simulink model "DYN_04"  (R2018b)
settings: Solver=FixedStepAuto  StartTime=0.0  StopTime=30  FixedStep=0.01  RelTol=1e-3
(part 1 of 14)
settings Model: Creator=TMP  LastModifiedBy=TMP
settings DataIOCC: ReturnWorkspaceOutputs=on

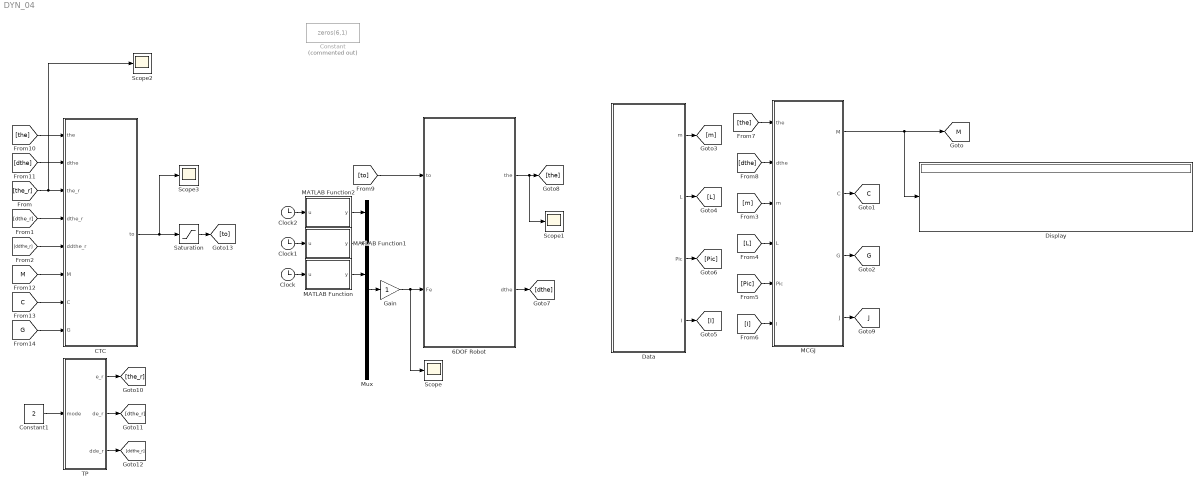
== system DYN_04 ==
  6DOF Robot : Subsystem
  CTC : MATLAB Function  TreatAsAtomicUnit=on
  Clock : Clock
  Clock1 : Clock
  Clock2 : Clock
  Constant : Constant  Commented=on  Value=zeros(6,1)
  Constant1 : Constant  Value=2
  Data : MATLAB Function  TreatAsAtomicUnit=on
  Display : Display
  Gain : Gain
  MATLAB Function : MATLAB Function  TreatAsAtomicUnit=on
  MATLAB Function1 : MATLAB Function  TreatAsAtomicUnit=on
  MATLAB Function2 : MATLAB Function  TreatAsAtomicUnit=on
  MCGJ : MATLAB Function  TreatAsAtomicUnit=on
  Mux : Mux  Inputs=6
  Saturation : Saturate  UpperLimit=500  LowerLimit=-500
  Scope{,1..3} (4 alike) : Scope
  TP : Subsystem
  tag scope: C=global, G=global, J=global, M=global
  wires:
  MCGJ/1(M) -> Display/1, [M]
  MCGJ/2(C) -> [C]
  MCGJ/3(G) -> [G]
  Data/1(m) -> [m]
  Data/2(L) -> [L]
  Data/3(Pic) -> [Pic]
  Data/4(I) -> [I]
  [L] -> MCGJ/4(L)
  [Pic] -> MCGJ/5(Pic)
  [I] -> MCGJ/6(I)
  [m] -> MCGJ/3(m)
  [dthe] -> MCGJ/2(dthe)
  [the] -> MCGJ/1(the)
  MCGJ/4(J) -> [J]
  6DOF Robot/1(the) -> Scope1/1, [the]
  6DOF Robot/2(dthe) -> [dthe]
  MATLAB Function/1(y) -> Mux/3
  Mux/1 -> Gain/1
  TP/1(e_r) -> [the_r]
  TP/2(de_r) -> [dthe_r]
  TP/3(dde_r) -> [ddthe_r]
  [the] -> CTC/1(the)
  [dthe] -> CTC/2(dthe)
  [the_r] -> Scope2/1, CTC/3(the_r)
  [dthe_r] -> CTC/4(dthe_r)
  [ddthe_r] -> CTC/5(ddthe_r)
  [M] -> CTC/6(M)
  [C] -> CTC/7(C)
  [G] -> CTC/8(G)
  Saturation/1 -> [to]
  Gain/1 -> Scope/1, 6DOF Robot/2(Fe)
  [to] -> 6DOF Robot/1(to)
  CTC/1(to) -> Scope3/1, Saturation/1
  Constant1/1 -> TP/1(mode)
  Clock/1 -> MATLAB Function/1(u)
  Clock1/1 -> MATLAB Function1/1(u)
  MATLAB Function1/1(y) -> Mux/2
  Clock2/1 -> MATLAB Function2/1(u)
  MATLAB Function2/1(y) -> Mux/1

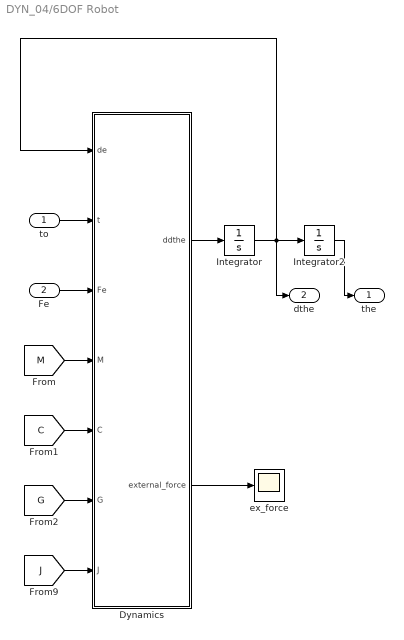
== system DYN_04/6DOF Robot ==
  to : Inport
  Fe : Inport  Port=2
  Dynamics : MATLAB Function  TreatAsAtomicUnit=on
  Integrator : Integrator  InitialCondition=[0;0;0;0;0;0]  UpperSaturationLimit=pi  LowerSaturationLimit=-pi
  Integrator2 : Integrator  InitialCondition=[0;0;0;0;0;0]  UpperSaturationLimit=[170;120;90;120;60;180]*pi/180  LowerSaturationLimit=-[170;120;90;120;60;180]*pi/180
  ex_force : Scope
  the : Outport
  dthe : Outport  Port=2
  wires:
  Integrator2/1 -> the/1
  Dynamics/1(ddthe) -> Integrator/1
  [C] -> Dynamics/5(C)
  [J] -> Dynamics/7(J)
  Integrator/1 -> Integrator2/1, Dynamics/1(de), dthe/1
  [M] -> Dynamics/4(M)
  [G] -> Dynamics/6(G)
  to/1 -> Dynamics/2(t)
  Dynamics/2(external_force) -> ex_force/1
  Fe/1 -> Dynamics/3(Fe)

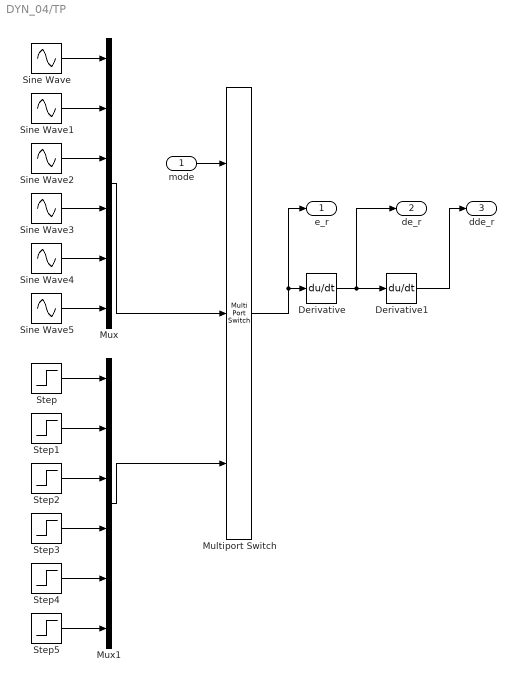
== system DYN_04/TP ==
  mode : Inport
  Derivative : Derivative
  Derivative1 : Derivative
  Multiport Switch : MultiPortSwitch  Inputs=2
  Mux : Mux  Inputs=6
  Mux1 : Mux  Inputs=6
  Sine Wave{,1..5} (6 alike) : Sin  Amplitude=pi/6  Frequency=2*pi*0.2  SampleTime=0
  Step{,1..5} (6 alike) : Step  After=0  SampleTime=0
  e_r : Outport
  de_r : Outport  Port=2
  dde_r : Outport  Port=3
  wires:
  Sine Wave/1 -> Mux/1
  Sine Wave1/1 -> Mux/2
  Sine Wave2/1 -> Mux/3
  Sine Wave3/1 -> Mux/4
  Sine Wave4/1 -> Mux/5
  Sine Wave5/1 -> Mux/6
  Mux/1 -> Multiport Switch/2
  Mux1/1 -> Multiport Switch/3
  Step2/1 -> Mux1/3
  Step5/1 -> Mux1/6
  Step1/1 -> Mux1/2
  Step3/1 -> Mux1/4
  Step/1 -> Mux1/1
  Step4/1 -> Mux1/5
  Multiport Switch/1 -> e_r/1, Derivative/1
  Derivative/1 -> de_r/1, Derivative1/1
  Derivative1/1 -> dde_r/1
  mode/1 -> Multiport Switch/1

== matlab function DYN_04/6DOF Robot/Dynamics ==
  data: de input; t input; Fe input; M input; ddthe output; C input; G input; J input; external_force output
function [ddthe,external_force] = DYN_6DOF(de,t,Fe,M,C,G,J)
%%
Fc = diag([0,0,0,0,0,0]);
Fv = 1*diag([5,5,5,0.5,0.1,0.05]);
external_force = Fc*sign(de) + Fv*de + J.'*Fe;
%%
ddthe = inv(M)*(t - C*de - G - external_force);
